simulink library "Lib_Turbo_Mixer_TMATS_org"  (Simulink 10.0)
settings: Solver=ode45  StartTime=0.0  StopTime=10.0  RelTol=1e-3  EnableMultiTasking=on
undefined symbols (not defined in the file): stripchar_TMATS
libraries: Lib_Solve_DataOut_TMATS x1
Description:
  | Thomas Modules
settings Model: Creator=jwchapm2  LastModifiedBy=bhisma

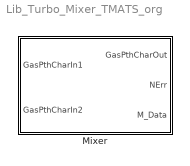
== system Lib_Turbo_Mixer_TMATS_org ==
  Mixer : Subsystem  mask(T-MATS: Mixer Library Block){Aphy1_M=10, Aphy2_M=10, s_M_Imp1_M=1, s_M_Imp2_M=1, s_M_V1_M=1, s_M_V2_M=1, Y_M_FARVec_M=[0; 0.0050; 0.0100; 0.0150; 0.0200; 0.0250; 0.0300], T_M_RtArray_M=[0.0686;    0.0686;    0.0686;    0.0686;    0.0686;    0.0686;    0.0686], X_M_TVec_M=[300 10000], T_M_gammaArray_M=[ 1.4 1.4 1.4 1.4 1.4 1.4 1.4; 1.4 1.4 1.4 1.4 1.4 1.4 1.4], iDesign_M=0, SWPS_M=0, BPRDes_M=0.5, MNDes_M=0.4, FVar_M=strcat('iDes_',stripchar_TMATS(gcb),'.bin')}
      mask prompts: Aphy1_M "Aphy1_M - Area of input 1 (in^2)"; Aphy2_M "Aphy2_M - Area of input 2 (in^2)"; s_M_Imp1_M "s_M_Imp1_M - Impulse 1 scalar"; s_M_Imp2_M "s_M_Imp2_M - Impulse 2 scalar"; s_M_V1_M "s_M_V1_M - Velocity 1 scalar"; s_M_V2_M "s_M_V2_M - Velocity 2 scalar"; Y_M_FARVec_M "Y_M_FARVec_M - Fuel to Air Ratio Vector (Y-axis)(cx1)"; T_M_RtArray_M "T_M_RtArray_M -  Rt Array (Rt = f(FAR))(cx1)"; X_M_TVec_M "X_M_TVec_M - Nozzle Total Temperature Vector (X-axis for Gamma calc)(dx1)"; T_M_gammaArray_M "T_M_gammaArray_M - Nozzle Map Gamma Array (Gamma = f(Tt,FAR))(dxc)"; iDesign_M "iDesign_M - Design fork (0 - Enable iDes, 1 - Use iDes Ath, 2 - Use Input Ath)"; SWPS_M "SWPS_M -  primary flow switch ( 0- primary flow is input 1, 1- primary flow is input 2)"; BPRDes_M "BPRDes_M -  Design bypass ratio [ W1/W2]"; MNDes_M "MNDes_M -  Primary flow Mach Number"; FVar_M "FVar_M - File name for iDes Variables"
      mask help: This block simulates the performance of a flow mixer using basic thermodynamic equations, properties, and table lookups.
      mask init:
      | if iDesign_M == 1
      |     P = load(FVar_M);
      |     Aphy1_M = P(1);
      |     Aphy2_M = P(2);
      | end
      mask Help: web(which('Turbo_TMATS_Mix.html'),'-helpbrowser')
      mask Callback iDesign_M:
      | MSK_SEC_Enables_Ides_TMATS('iDesign_M',[1 2],'G1')
      | MSK_SEC_Enables_Ides_TMATS('iDesign_M',[12 13 14],'G2')
      | MSK_SEC_Enables_Ides_TMATS('iDesign_M',[15],'G3')

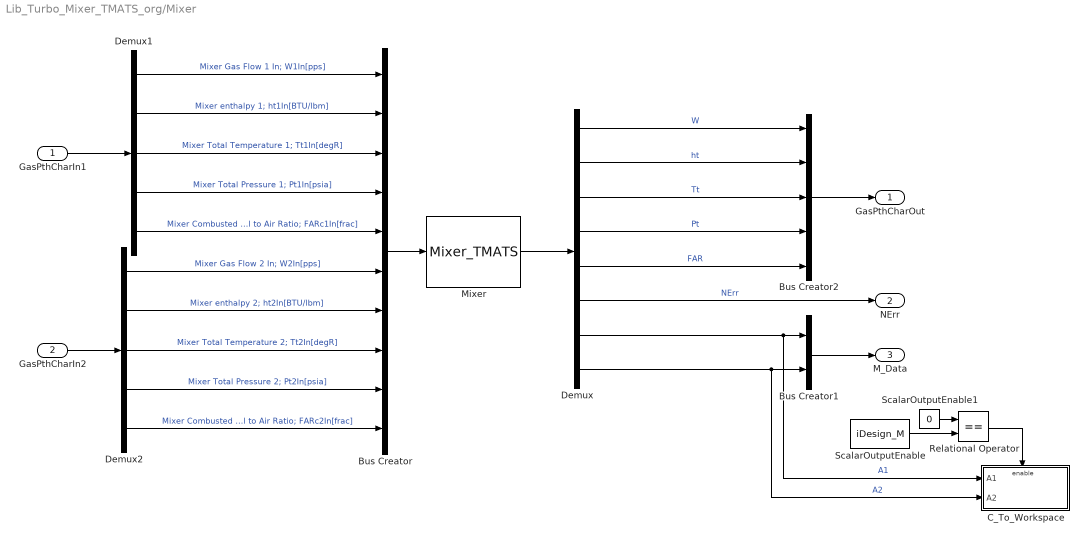
== system Lib_Turbo_Mixer_TMATS_org/Mixer ==
  GasPthCharIn1 : Inport
  GasPthCharIn2 : Inport  Port=2
  Bus Creator : BusCreator  Inputs=10
  Bus Creator1 : BusCreator  Inputs=2
  Bus Creator2 : BusCreator  Inputs=5
  C_To_Workspace : Subsystem
  Demux : Demux  Outputs=8
  Demux1 : Demux  Outputs=5
  Demux2 : Demux  Outputs=5
  Mixer : S-Function  FunctionName=Mixer_TMATS  Parameters=Aphy1_M, Aphy2_M, Y_M_FARVec_M, X_M_TVec_M, T_M_RtArray_M, T_M_gammaArray_M, s_M_Imp1_M, s_M_Imp2_M, s_M_V1_M, s_M_V2_M, iDesign_M, SWPS_M, BPRDes_M, MNDes_M, gcs  SFunctionModules='t2hc_TMATS h2tc_TMATS pt2sc_TMATS sp2tc_TMATS interp1Ac_TMATS interp2Ac_TMATS PcalcStat_TMATS functions_TMATS'  SFunctionDeploymentMode=off  EnableBusSupport=off
  Relational Operator : RelationalOperator  Operator===  OutDataTypeStr=boolean  RndMeth=Nearest
  ScalarOutputEnable : Constant  Value=iDesign_M
  ScalarOutputEnable1 : Constant  Value=0
  GasPthCharOut : Outport
  NErr : Outport  Port=2
  M_Data : Outport  Port=3
  wires:
  Demux1/4 -> Bus Creator/4  "Mixer Total Pressure 1; Pt1In[psia]"
  Bus Creator/1 -> Mixer/1
  Demux/4 -> Bus Creator2/4  "Pt"
  Demux/3 -> Bus Creator2/3  "Tt"
  Demux/5 -> Bus Creator2/5  "FAR"
  Demux/1 -> Bus Creator2/1  "W"
  Mixer/1 -> Demux/1
  Demux1/3 -> Bus Creator/3  "Mixer Total Temperature 1; Tt1In[degR]"
  Demux1/5 -> Bus Creator/5  "Mixer Combusted Fuel to Air Ratio; FARc1In[frac]"
  Demux/2 -> Bus Creator2/2  "ht"
  Bus Creator2/1 -> GasPthCharOut/1
  GasPthCharIn1/1 -> Demux1/1
  Demux1/1 -> Bus Creator/1  "Mixer Gas Flow 1 In; W1In[pps]"
  Demux1/2 -> Bus Creator/2  "Mixer enthalpy 1; ht1In[BTU/lbm]"
  Demux2/1 -> Bus Creator/6  "Mixer Gas Flow 2 In; W2In[pps]"
  Demux2/2 -> Bus Creator/7  "Mixer enthalpy 2; ht2In[BTU/lbm]"
  Demux2/3 -> Bus Creator/8  "Mixer Total Temperature 2; Tt2In[degR]"
  GasPthCharIn2/1 -> Demux2/1
  Demux2/4 -> Bus Creator/9  "Mixer Total Pressure 2; Pt2In[psia]"
  Demux2/5 -> Bus Creator/10  "Mixer Combusted Fuel to Air Ratio; FARc2In[frac]"
  Demux/6 -> NErr/1  "NErr"
  Demux/8 -> C_To_Workspace/2(A2), Bus Creator1/2  "A2"
  Demux/7 -> Bus Creator1/1, C_To_Workspace/1(A1)  "A1"
  ScalarOutputEnable/1 -> Relational Operator/2
  ScalarOutputEnable1/1 -> Relational Operator/1
  Relational Operator/1 -> C_To_Workspace/Enable
  Bus Creator1/1 -> M_Data/1

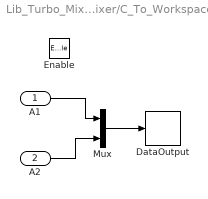
== system Lib_Turbo_Mixer_TMATS_org/Mixer/C_To_Workspace ==
  A1 : Inport
  A2 : Inport  Port=2
  Enable : EnablePort
  DataOutput : Lib_Solve_DataOut_TMATS/DataOutput  FVar_M=FVar_M
  Mux : Mux  Inputs=2
  wires:
  A1/1 -> Mux/1
  A2/1 -> Mux/2
  Mux/1 -> DataOutput/1
